simulink model "linear"  (R2021b)
settings: Solver=VariableStepAuto  StartTime=0.0  StopTime=10  RelTol=1e-3
values from neighbouring files (symbols this model uses):
  b = 0.02    [parameter.m]
  g = 9.81    [parameter.m]
  I = 1    [parameter.m]
  kv = 0.02    [parameter.m]
  L = 1.0    (= 1)    [parameter.m]
  M = 6.0    (= 6)    [parameter.m]
  m = 1.5    [parameter.m]
settings Model: Creator=Tolga Catak  LastModifiedBy=Tolga Catak

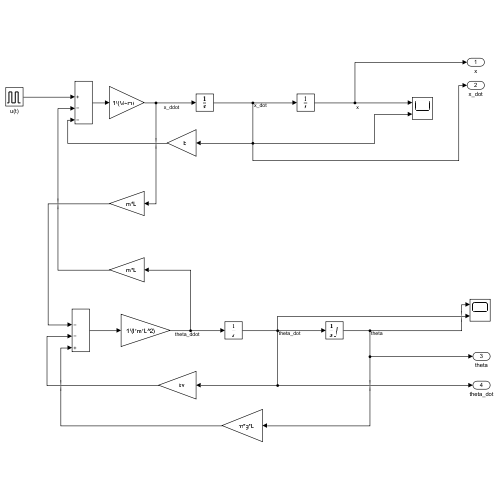
[thumbnail: Simulink's stored preview of the top-level diagram]
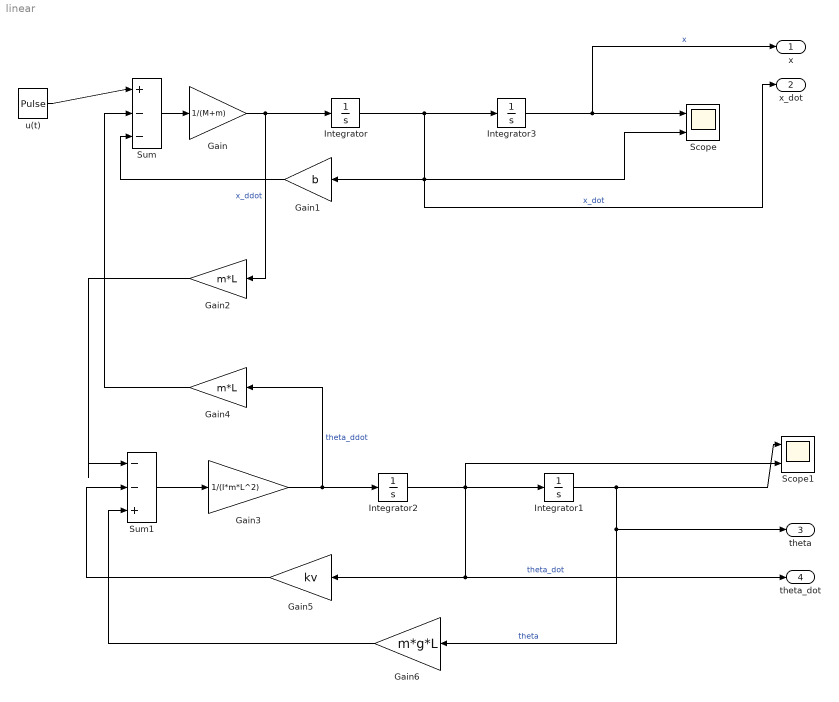
== system linear ==
  Gain : Gain  Gain=1/(M+m)
  Gain1 : Gain  Gain=b
  Gain2 : Gain  Gain=m*L
  Gain3 : Gain  Gain=1/(I*m*L^2)
  Gain4 : Gain  Gain=m*L
  Gain5 : Gain  Gain=kv
  Gain6 : Gain  Gain=m*g*L
  Integrator : Integrator
  Integrator1 : Integrator  LimitOutput=on
  Integrator2 : Integrator
  Integrator3 : Integrator
  Scope : Scope  NumInputPorts=2
  Scope1 : Scope  NumInputPorts=2
  Sum : Sum  Inputs=|+--
  Sum1 : Sum  Inputs=|--+
  "u(t) " : DiscretePulseGenerator  PulseType=Time based  Amplitude=100  Period=10  PulseWidth=0.01
  x : Outport
  x_dot : Outport  Port=2
  theta : Outport  Port=3
  theta_dot : Outport  Port=4
  wires:
  "u(t) "/1 -> Sum/1
  Gain3/1 -> Gain4/1, Integrator2/1  "theta_ddot"
  Gain4/1 -> Sum/2
  Sum1/1 -> Gain3/1
  Gain6/1 -> Sum1/3
  Gain5/1 -> Sum1/2
  Integrator1/1 -> theta/1, Gain6/1, Scope1/1  "theta"
  Gain2/1 -> Sum1/1
  Integrator3/1 -> Scope/1, x/1  "x"
  Sum/1 -> Gain/1
  Gain1/1 -> Sum/3
  Gain/1 -> Gain2/1, Integrator/1  "x_ddot"
  Integrator/1 -> Gain1/1, x_dot/1, Scope/2, Integrator3/1  "x_dot"
  Integrator2/1 -> Integrator1/1, Scope1/2, theta_dot/1, Gain5/1  "theta_dot"
